simulink model "Bicopter_Dynamics"  (R2019a)
settings: Solver=ode4  StartTime=0.0  StopTime=25  FixedStep=0.0001  RelTol=1e-3
undefined symbols (not defined in the file or in its folder): sigbuilder_block
settings Model: Creator=crsmyth  LastModifiedBy=crs20

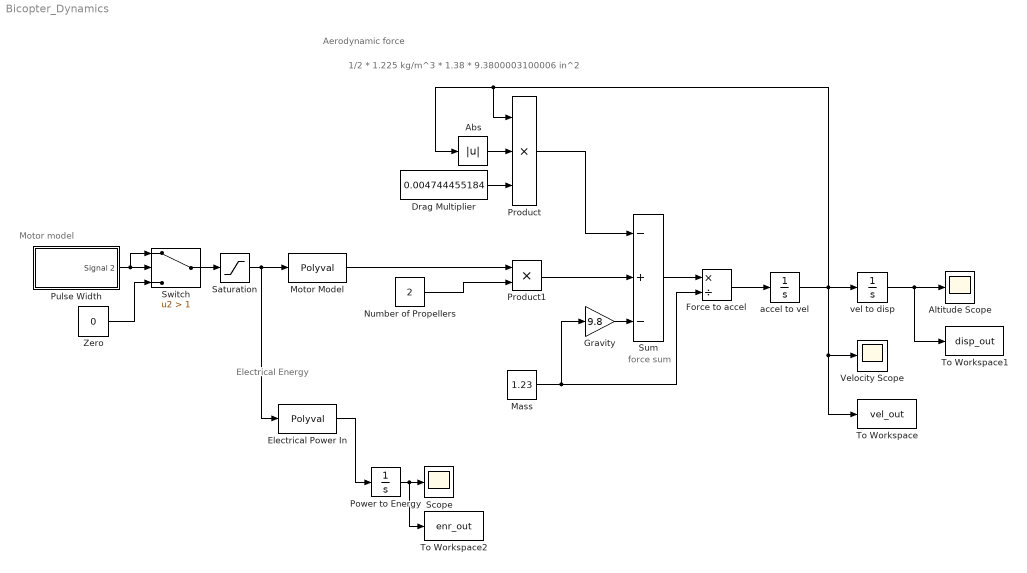
== system Bicopter_Dynamics ==
  note: Electrical Energy
  note: force sum
  note: Motor model
  note: Aerodynamic force
  note: 1/2 * 1.225 kg/m^3 * 1.38 * 9.3800003100006 in^2
  Abs : Abs
  Altitude Scope : Scope
  Drag Multiplier : Constant  Value=0.004744455184
  Electrical Power In : Polyval  Coefs=[2.956191832898671e+02, -6.235353126465623e+02, 3.330393150826374e+02]
  Force to accel : Product  Inputs=*/
  Gravity : Gain  Gain=9.8
  Mass : Constant  Value=1.23
  Motor Model : Polyval  Coefs=[4.843819998761814,-4.792311105872948,-0.068689974553541]
  Number of Propellers : Constant  Value=2
  Power to Energy : Integrator
  Product : Product  Inputs=3
  Product1 : Product
  Pulse Width : Subsystem  Tag=STV Subsys  LoadFcn=sigbuilder_block('load');  StartFcn=sigbuilder_block('start');  StopFcn=sigbuilder_block('stop');  ClipboardFcn=sigbuilder_block('clipboard');  mask(Sigbuilder block){tuvar=[0:10]}
      mask help: Simulink:masks:SigbuilderBlock_MD
      mask init:
      | if ~strcmp(get_param(bdroot(gcbh),'SimulationStatus'),'stopped') tuvar = sigbuilder_block('maskInit'); end
      settings: CopyFcn=sigbuilder_block('copy');  DeleteFcn=sigbuilder_block('delete');  ModelCloseFcn=sigbuilder_block('modelClose');  PreSaveFcn=sigbuilder_block('preSave');  PauseFcn=sigbuilder_block('pause');  ContinueFcn=sigbuilder_block('continue');  NameChangeFcn=sigbuilder_block('namechange');  OpenFcn=sigbuilder_block('open',[261 219.75 550.5 360.75 ]);  CloseFcn=sigbuilder_block('close');
      mask Display: plot(0, 0, 100, 100,[2, 2, 32, 32, 2], [68, 8, 8, 68, 68],[32, 2], [38, 38], [32, 19, 2],[53, 60, 44], [32, 17, 17, 2],[16, 16, 31, 31]);txt = getActiveGroup(gcbh);text(2, 100, txt,'verticalAlignment', 'top');
  Saturation : Saturate  UpperLimit=2  LowerLimit=0
  Scope : Scope
  Sum : Sum  Inputs=-+-
  Switch : Switch  Criteria=u2 > Threshold  Threshold=1
  To Workspace : ToWorkspace  VariableName=vel_out  SampleTime=-1
      settings: Save2DSignal=2-D array (concatenate along first dimension)
  To Workspace1 : ToWorkspace  VariableName=disp_out  SampleTime=-1
      settings: Save2DSignal=2-D array (concatenate along first dimension)
  To Workspace2 : ToWorkspace  VariableName=enr_out  SaveFormat=Timeseries  SampleTime=-1
  Velocity Scope : Scope
  Zero : Constant  Value=0  OutDataTypeStr=Inherit: Inherit via back propagation
  accel to vel : Integrator
  vel to disp : Integrator
  wires:
  Sum/1 -> Force to accel/1
  Mass/1 -> Gravity/1, Force to accel/2
  Force to accel/1 -> accel to vel/1
  Gravity/1 -> Sum/3
  Product/1 -> Sum/1
  Drag Multiplier/1 -> Product/3
  Abs/1 -> Product/2
  Product1/1 -> Sum/2
  Number of Propellers/1 -> Product1/2
  Motor Model/1 -> Product1/1
  accel to vel/1 -> vel to disp/1, Abs/1, Product/1, To Workspace/1, Velocity Scope/1
  vel to disp/1 -> To Workspace1/1, Altitude Scope/1
  Electrical Power In/1 -> Power to Energy/1
  Power to Energy/1 -> To Workspace2/1, Scope/1
  Saturation/1 -> Electrical Power In/1, Motor Model/1
  Pulse Width/1(Signal 2) -> Switch/1, Switch/2
  Zero/1 -> Switch/3
  Switch/1 -> Saturation/1

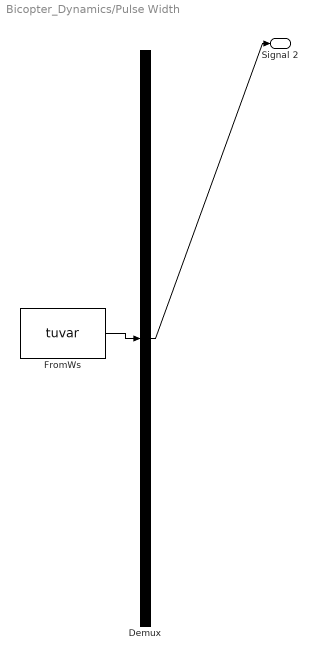
== system Bicopter_Dynamics/Pulse Width ==
  Demux : Demux  Tag=STV Demux  Outputs=1
  FromWs : FromWorkspace  Tag=STV FromWs  VariableName=tuvar  SampleTime=0
      SigBuilderData=|
      | common.afterFinalStr = 'Extrapolate'
      | common.sampleTime = 0
      | dataSet.timeRange = [0 25]
      | dataSet.name = 'Group 1'
      | sbobj.Groups.Name = 'Group 1'
      | sbobj.Groups.Signals.Name = 'Signal 2'
      | sbobj.Groups.Signals.XData = [0 4.95 4.95 7.305 7.305 13.3 13.3 16.4 16.4 20.391 20.391 25]
      | sbobj.Groups.Signals.YData = [2 2 1 1 1.72072 1.72072 1 1 2 2 1.7207 1.7207]
      | sbobj.Groups.TimeRange = [0 25]
  Signal 2 : Outport  Tag=STV Outport
  wires:
  FromWs/1 -> Demux/1
  Demux/1 -> Signal 2/1
